simulink model "Expt_5_2"  (R2018b)
settings: Solver=VariableStepAuto  StartTime=0.0  StopTime=10.0  RelTol=1e-3
libraries: simulink x1
settings Model: Creator=HP  LastModifiedBy=HP
settings DebuggingCC: LibraryContextMissingDiagnostic=none
settings SFSimCC: SimUseLocalCustomCode=off
settings RTWCC: RTWUseLocalCustomCode=off

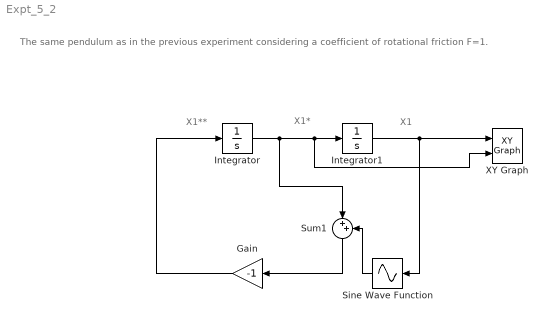
== system Expt_5_2 ==
  note: X1
  note: X1*
  note: X1**
  note: The same pendulum as in the previous experiment considering a coefficient of rotational friction F=1.
  Gain : Gain  Gain=-1
  Integrator : Integrator  InitialCondition=1
  Integrator1 : Integrator  InitialCondition=-3.2
  Sine Wave Function : Sin  TimeSource=Use external signal  SampleTime=0
  Sum1 : Sum  Inputs=|++
  XY Graph : simulink/Sinks/XY Graph  xmin=-10  xmax=10  ymin=-10  ymax=10  st=-1
  wires:
  Integrator1/1 -> Sine Wave Function/1, XY Graph/1
  Integrator/1 -> Sum1/1, XY Graph/2, Integrator1/1
  Gain/1 -> Integrator/1
  Sum1/1 -> Gain/1
  Sine Wave Function/1 -> Sum1/2
